simulink model "DualEMDriveRear4EMSSC"  (R2026b)
settings: Solver=VariableStepAuto
undefined symbols (not defined in the file): AxlRL, AxlRR, DriveshftTrq3, DriveshftTrq4, PlntEMWhlGearInDampRL, PlntEMWhlGearInDampRR, PlntEMWhlGearOutDampRL, PlntEMWhlGearOutDampRR
libraries: fl_lib x4, sdl_lib x2
settings Model: ModifiedByFormat=The MathWorks, Inc.  Creator=The MathWorks, Inc.  LastModifiedBy=The MathWorks, Inc.
settings OptimizationCC: ReuseModelBlockBuffer=off
settings SimscapeCC: SimscapeUseEnergyAccounting=off

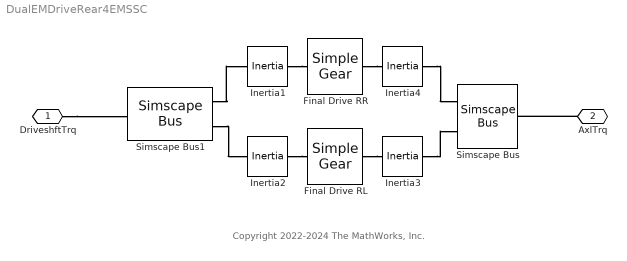
== system DualEMDriveRear4EMSSC ==
  note: Copyright 2022-2024 The MathWorks, Inc.
  Final Drive RL : sdl_lib/Gears/Simple Gear  ratio=PlntEMWhlGearRatioRL  rotation_direction=sdl.enum.shaftOutputDirection.same  friction_model=sdl.enum.gear_efficiencies_load.constant  T_noload=0.1 N*m  T_nom=5 N*m  efficiency_nom=0.8  efficiency=PlntEMWhlGearEffRL  temperature_TLU=[280, 300, 320] K  load_TLU=[1, 5, 10] N*m  efficiency_TLU=[.95, .9, .85]  efficiency_TLU2=[.85, .8, .75; .95, .9, .85; .85, .8, .7]  w_thr=0.01 rad/s  pwr_thr=PlntEMWhlGearRLPwrThresh W  enable_backlash=false  hardstop_model=simscape.enum.hardstop.smooth  backlash_distance=1e-3 mm  r_base=0.1 m  transition=1e-4 mm  backlash_stiffness=1e7 N/m  backlash_damping=1e6 N*s/m  coeff_rest=0  v_tol=0.001 m/s  f_tol=0 N  tau=0.1 s  mu_visc=[PlntEMWhlGearInDampRL PlntEMWhlGearOutDampRL] N*m*s/rad  thermal_mass=50 J/K  temperature_specify=off  temperature_priority=High  temperature=300 K  temperature_nominal_specify=off  temperature_nominal_value=1  temperature_nominal_unit=K  x_backlash_specify=off  x_backlash_priority=None  x_backlash=0 mm  x_backlash_nominal_specify=off  x_backlash_nominal_value=1  x_backlash_nominal_unit=mm  f_hardstop_specify=off  f_hardstop_priority=None  f_hardstop=0 N  f_hardstop_nominal_specify=off  f_hardstop_nominal_value=1  f_hardstop_nominal_unit=N  v_backlash_specify=off  v_backlash_priority=None  v_backlash=0 m/s  v_backlash_nominal_specify=off  v_backlash_nominal_value=1  v_backlash_nominal_unit=m/s
  Final Drive RR : sdl_lib/Gears/Simple Gear  ratio=PlntEMWhlGearRatioRR  rotation_direction=sdl.enum.shaftOutputDirection.same  friction_model=sdl.enum.gear_efficiencies_load.constant  T_noload=0.1 N*m  T_nom=5 N*m  efficiency_nom=0.8  efficiency=PlntEMWhlGearEffRR  temperature_TLU=[280, 300, 320] K  load_TLU=[1, 5, 10] N*m  efficiency_TLU=[.95, .9, .85]  efficiency_TLU2=[.85, .8, .75; .95, .9, .85; .85, .8, .7]  w_thr=0.01 rad/s  pwr_thr=PlntEMWhlGearRRPwrThresh W  enable_backlash=false  hardstop_model=simscape.enum.hardstop.smooth  backlash_distance=1e-3 mm  r_base=0.1 m  transition=1e-4 mm  backlash_stiffness=1e7 N/m  backlash_damping=1e6 N*s/m  coeff_rest=0  v_tol=0.001 m/s  f_tol=0 N  tau=0.1 s  mu_visc=[PlntEMWhlGearInDampRR PlntEMWhlGearOutDampRR] N*m*s/rad  thermal_mass=50 J/K  temperature_specify=off  temperature_priority=High  temperature=300 K  temperature_nominal_specify=off  temperature_nominal_value=1  temperature_nominal_unit=K  x_backlash_specify=off  x_backlash_priority=None  x_backlash=0 mm  x_backlash_nominal_specify=off  x_backlash_nominal_value=1  x_backlash_nominal_unit=mm  f_hardstop_specify=off  f_hardstop_priority=None  f_hardstop=0 N  f_hardstop_nominal_specify=off  f_hardstop_nominal_value=1  f_hardstop_nominal_unit=N  v_backlash_specify=off  v_backlash_priority=None  v_backlash=0 m/s  v_backlash_nominal_specify=off  v_backlash_nominal_value=1  v_backlash_nominal_unit=m/s
  Inertia1 : fl_lib/Mechanical/Rotational Elements/Inertia  inertia=PlntEMWhlGearInInertiaRR kg*m^2  num_ports=foundation.enum.numPorts2.two  w_specify=off  w_priority=High  w=0 rad/s  w_nominal_specify=off  w_nominal_value=1  w_nominal_unit=rad/s  t_specify=off  t_priority=None  t=0 N*m  t_nominal_specify=off  t_nominal_value=1  t_nominal_unit=N*m
  Inertia2 : fl_lib/Mechanical/Rotational Elements/Inertia  inertia=PlntEMWhlGearInInertiaRL kg*m^2  num_ports=foundation.enum.numPorts2.two  w_specify=off  w_priority=High  w=0 rad/s  w_nominal_specify=off  w_nominal_value=1  w_nominal_unit=rad/s  t_specify=off  t_priority=None  t=0 N*m  t_nominal_specify=off  t_nominal_value=1  t_nominal_unit=N*m
  Inertia3 : fl_lib/Mechanical/Rotational Elements/Inertia  inertia=PlntEMWhlGearOutInertiaRL kg*m^2  num_ports=foundation.enum.numPorts2.two  w_specify=off  w_priority=High  w=0 rad/s  w_nominal_specify=off  w_nominal_value=1  w_nominal_unit=rad/s  t_specify=off  t_priority=None  t=0 N*m  t_nominal_specify=off  t_nominal_value=1  t_nominal_unit=N*m
  Inertia4 : fl_lib/Mechanical/Rotational Elements/Inertia  inertia=PlntEMWhlGearOutInertiaRR kg*m^2  num_ports=foundation.enum.numPorts2.two  w_specify=off  w_priority=High  w=0 rad/s  w_nominal_specify=off  w_nominal_value=1  w_nominal_unit=rad/s  t_specify=off  t_priority=None  t=0 N*m  t_nominal_specify=off  t_nominal_value=1  t_nominal_unit=N*m
  Simscape Bus : SimscapeBus  HierarchyStrings=AxlRR;AxlRL
  Simscape Bus1 : SimscapeBus  HierarchyStrings=DriveshftTrq4;DriveshftTrq3
  DriveshftTrq : PMIOPort  Side=Left
  AxlTrq : PMIOPort  Port=2  Side=Right
  connections:
  DriveshftTrq/RConn1 -- Simscape Bus1/RConn1
  AxlTrq/RConn1 -- Simscape Bus/RConn1
  Inertia4/LConn1 -- Simscape Bus/LConn1
  Simscape Bus1/LConn1 -- Inertia1/RConn1
  Final Drive RR/RConn1 -- Inertia4/RConn1
  Inertia1/LConn1 -- Final Drive RR/LConn1
  Inertia2/LConn1 -- Final Drive RL/LConn1
  Inertia3/LConn1 -- Simscape Bus/LConn2
  Final Drive RL/RConn1 -- Inertia3/RConn1
  Simscape Bus1/LConn2 -- Inertia2/RConn1
